simulink model "FilterModel"  (R2023a)
settings: Solver=VariableStepAuto  StartTime=0.0  StopTime=.1  RelTol=1e-9
model workspace (MAT data in the model file):
  omegac = 9424.77796077
settings Model: Creator=mcconncm  LastModifiedBy=mcconncm

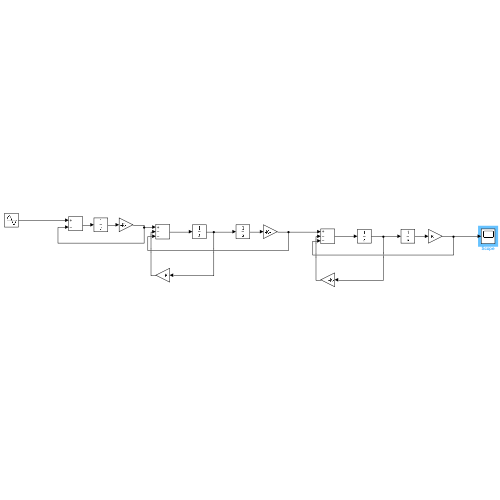
[thumbnail: Simulink's stored preview of the top-level diagram]
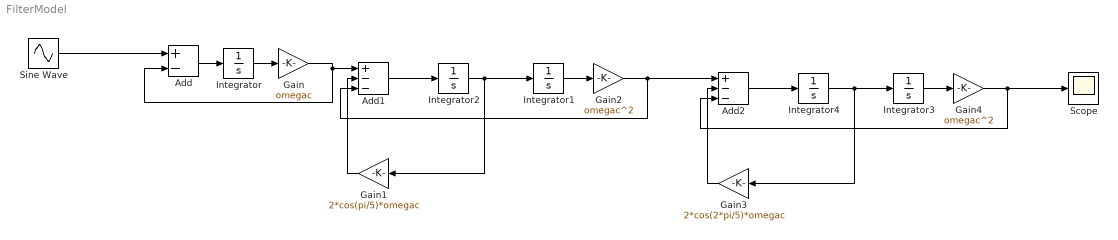
== system FilterModel ==
  Add : Sum  Inputs=+-
  Add1 : Sum  Inputs=+--
  Add2 : Sum  Inputs=+--
  Gain : Gain  Gain=omegac
  Gain1 : Gain  Gain=2*cos(pi/5)*omegac
  Gain2 : Gain  Gain=omegac^2
  Gain3 : Gain  Gain=2*cos(2*pi/5)*omegac
  Gain4 : Gain  Gain=omegac^2
  Integrator{,1..4} (5 alike) : Integrator
  Scope : Scope
  Sine Wave : Sin  Frequency=1000*2*pi  SampleTime=0
  wires:
  Add/1 -> Integrator/1
  Integrator/1 -> Gain/1
  Gain/1 -> Add1/1, Add/2
  Add1/1 -> Integrator2/1
  Integrator2/1 -> Gain1/1, Integrator1/1
  Gain1/1 -> Add1/2
  Integrator1/1 -> Gain2/1
  Add2/1 -> Integrator4/1
  Gain3/1 -> Add2/2
  Integrator3/1 -> Gain4/1
  Gain4/1 -> Scope/1, Add2/3
  Integrator4/1 -> Gain3/1, Integrator3/1
  Gain2/1 -> Add2/1, Add1/3
  Sine Wave/1 -> Add/1
